simulink model "Eg3_5"  (R2018a)
settings: Solver=VariableStepAuto  StartTime=0.0  StopTime=10.0  RelTol=1e-3
settings Model: Creator=wangluo  LastModifiedBy=wangluo

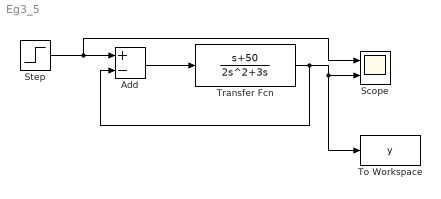
== system Eg3_5 ==
  Add : Sum  Inputs=+-
  Scope : Scope  NumInputPorts=2
  Step : Step  SampleTime=0
  To Workspace : ToWorkspace  VariableName=y  SampleTime=-1
  Transfer Fcn : TransferFcn  Numerator=[1 50]  Denominator=[2 3 0]
  wires:
  Add/1 -> Transfer Fcn/1
  Transfer Fcn/1 -> Add/2, To Workspace/1, Scope/2
  Step/1 -> Add/1, Scope/1
